simulink subsystem "ctrl_mngr_sub"  (R2024b)
settings: Solver=VariableStepAuto  StartTime=0.0  StopTime=10.0  RelTol=1e-3
settings Model: Creator=Angel  LastModifiedBy=Angel

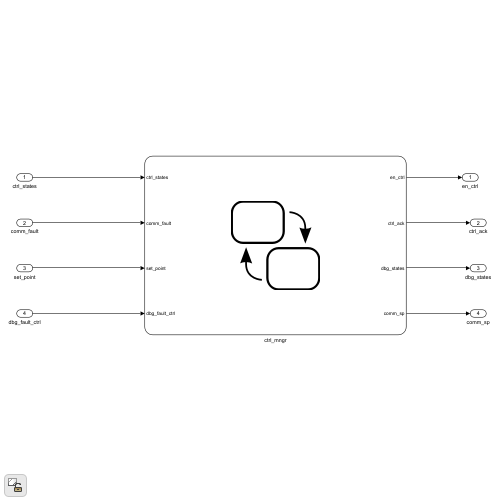
[thumbnail: Simulink's stored preview of the top-level diagram]
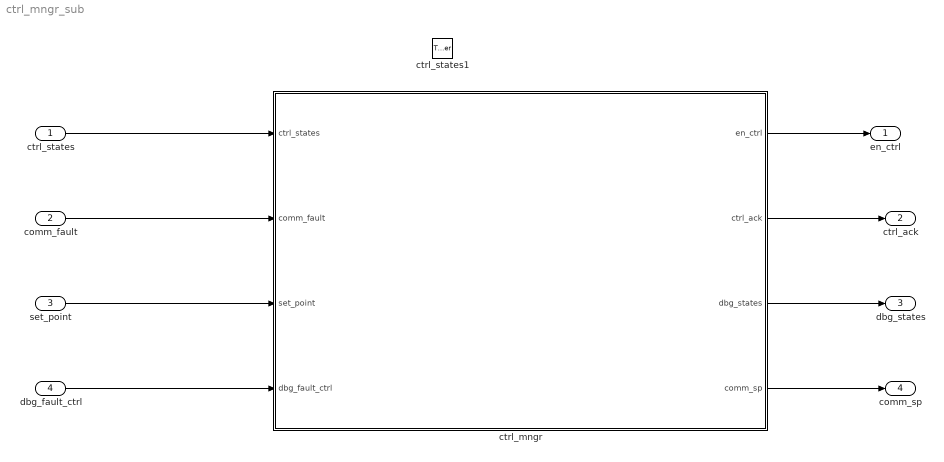
== system ctrl_mngr_sub ==
  ctrl_states : Inport
  comm_fault : Inport  Port=2
  set_point : Inport  Port=3
  dbg_fault_ctrl : Inport  Port=4
  ctrl_states1 : TriggerPort  TriggerType=function-call  VariantControl=(inherit)  PortDimensions=1
  ctrl_mngr : Stateflow chart  TreatAsAtomicUnit=on
  en_ctrl : Outport
  ctrl_ack : Outport  Port=2
  dbg_states : Outport  Port=3
  comm_sp : Outport  Port=4
  wires:
  ctrl_mngr/2(ctrl_ack) -> ctrl_ack/1
  ctrl_mngr/1(en_ctrl) -> en_ctrl/1
  set_point/1 -> ctrl_mngr/3(set_point)
  ctrl_mngr/4(comm_sp) -> comm_sp/1
  dbg_fault_ctrl/1 -> ctrl_mngr/4(dbg_fault_ctrl)
  ctrl_states/1 -> ctrl_mngr/1(ctrl_states)
  ctrl_mngr/3(dbg_states) -> dbg_states/1
  comm_fault/1 -> ctrl_mngr/2(comm_fault)

== stateflow chart ctrl_mngr_sub/ctrl_mngr ==
  state off
    en:
    en_ctrl=false;
    ctrl_ack=00;
    dbg_states = 00;
    comm_sp=0;
  state on
    en:
    en_ctrl=true;
    ctrl_ack=01;
    dbg_states = 01;
    comm_sp=set_point;
  (default) -> off
  (junction 19) -> off
  (junction 18) -> (junction 19)
  off -> (junction 14)
  (junction 14) -> (junction 18) [order 1] : [comm_fault|dbg_fault_ctrl]
  (junction 26) -> (junction 18)
  (junction 14) -> on [order 2] : [ctrl_states==01]
  on -> (junction 24)
  (junction 24) -> (junction 26) [order 2] : [ctrl_states==00]
  (junction 31) -> (junction 26)
  (junction 24) -> (junction 29) [order 1]
  (junction 29) -> (junction 31) : [comm_fault|dbg_fault_ctrl]
  data: ctrl_states input uint8; comm_fault input boolean; set_point input single; dbg_fault_ctrl input boolean; en_ctrl output boolean; ctrl_ack output uint8; dbg_states output uint8; comm_sp output single
